simulink model "h4"  (R2019a)
settings: Solver=VariableStepAuto  StartTime=0.0  StopTime=30.0  MaxStep=0.003  MinStep=0.001  RelTol=1e-3
settings Model: Creator=toshiba1000  LastModifiedBy=toshiba1000
settings SolverCC: InitialStep=0.002

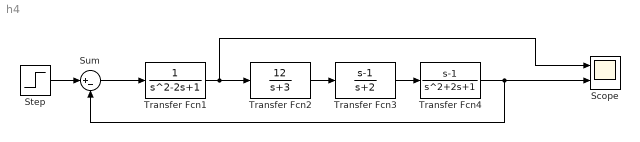
== system h4 ==
  Scope : Scope  NumInputPorts=2
  Step : Step  SampleTime=0
  Sum : Sum  Inputs=|+-
  Transfer Fcn1 : TransferFcn  Denominator=[1 -2 1]
  Transfer Fcn2 : TransferFcn  Numerator=[12]  Denominator=[1 3]
  Transfer Fcn3 : TransferFcn  Numerator=[1 -1]  Denominator=[1 2]
  Transfer Fcn4 : TransferFcn  Numerator=[1 -1]
  wires:
  Transfer Fcn2/1 -> Transfer Fcn3/1
  Transfer Fcn3/1 -> Transfer Fcn4/1
  Transfer Fcn4/1 -> Scope/2, Sum/2
  Transfer Fcn1/1 -> Scope/1, Transfer Fcn2/1
  Step/1 -> Sum/1
  Sum/1 -> Transfer Fcn1/1
